simulink model "timesFive"  (R2016b)
settings: Solver=VariableStepAuto  StartTime=0.0  StopTime=10.0  RelTol=1e-3
settings Model: Creator=Borja Martos  LastModifiedBy=Borja Martos

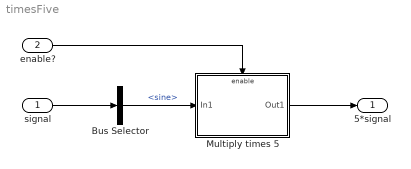
== system timesFive ==
  signal : Inport  OutDataTypeStr=Bus: slBus1
  enable? : Inport  Port=2
  Bus Selector : BusSelector  OutputSignals=sine
  Multiply times 5 : Subsystem
  5*signal : Outport
  wires:
  Multiply times 5/1(Out1) -> 5*signal/1
  enable?/1 -> Multiply times 5/Enable
  signal/1 -> Bus Selector/1
  Bus Selector/1 -> Multiply times 5/1(In1)  "<sine>"

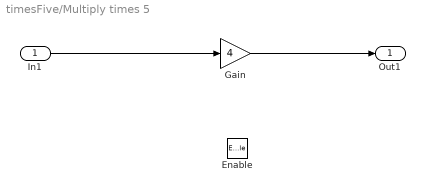
== system timesFive/Multiply times 5 ==
  In1 : Inport
  Enable : EnablePort  StatesWhenEnabling=reset
  Gain : Gain  Gain=4
  Out1 : Outport
  wires:
  Gain/1 -> Out1/1
  In1/1 -> Gain/1
